simulink model "fault_predictor"  (R2024b)
settings: Solver=FixedStepDiscrete  StartTime=0.0  StopTime=T_stop  FixedStep=0.1  RelTol=1e-3
undefined symbols (not defined in the file): fp_thresholds
settings Model: Creator=rayen  LastModifiedBy=rayen
settings OptimizationCC: DefaultParameterBehavior=Inlined  EnhancedBackFolding=on  PassReuseOutputArgsAs=Individual arguments  ZeroExternalMemoryAtStartup=off  ZeroInternalMemoryAtStartup=off  OptimizeBlockOrder=speed  DifferentSizesBufferReuse=on  OptimizationCustomize=off  EfficientTunableParamExpr=on
settings DebuggingCC: ParameterTunabilityLossMsg=error
settings HardwareCC: TargetBitPerPointer=64  TargetBitPerSizeT=64  TargetBitPerPtrDiffT=64  TargetLargestAtomicFloat=Float  TargetIntDivRoundTo=Zero  TargetEndianess=LittleEndian  TargetWordSize=64  TargetHWDeviceType=Intel->x86-64 (Windows64)  ProdEqTarget=off
settings SFSimCC: MATLABDynamicMemAlloc=off  SimTargetLang=C++
settings RTWCC: Description=Embedded Coder  SystemTargetFile=ert.tlc  TemplateMakefile=ert_default_tmf
settings CodeAppCC: ForceParamTrailComments=on  IgnoreCustomStorageClasses=off  OperatorAnnotations=on  SimulinkDataObjDesc=on  SFDataObjDesc=on  InsertBlockDesc=on
settings ERTTargetCC: TargetLangStandard=C99 (ISO)  GenerateSampleERTMain=on  ERTCustomFileTemplate=example_file_process.tlc

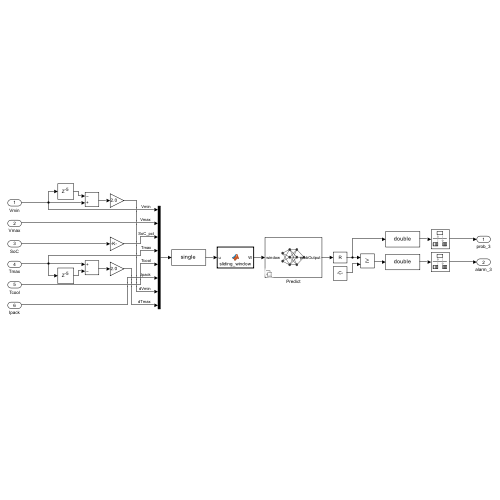
[thumbnail: Simulink's stored preview of the top-level diagram]
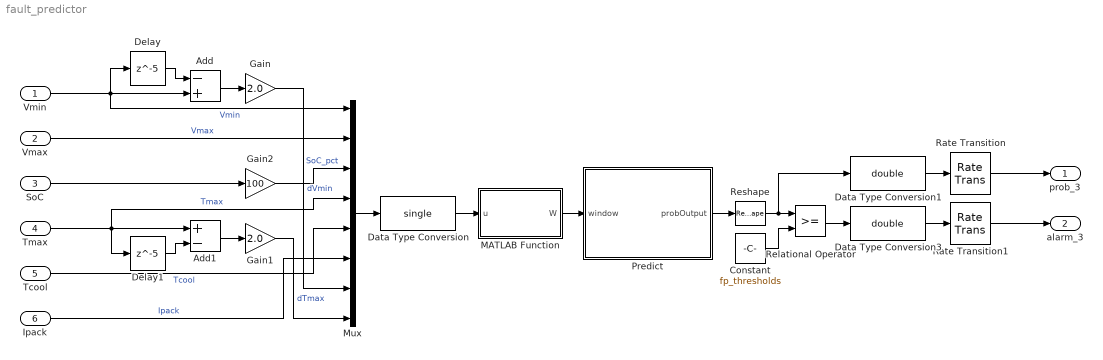
== system fault_predictor ==
  Vmin : Inport  SampleTime=0.1
  Vmax : Inport  Port=2  SampleTime=0.1
  SoC : Inport  Port=3  SampleTime=0.1
  Tmax : Inport  Port=4  SampleTime=0.1
  Tcool : Inport  Port=5  SampleTime=0.1
  Ipack : Inport  Port=6  SampleTime=0.1
  Add : Sum  Inputs=-+
  Add1 : Sum  Inputs=+-
  Constant : Constant  Value=fp_thresholds  OutDataTypeStr=single
  Data Type Conversion : DataTypeConversion  OutDataTypeStr=single  SaturateOnIntegerOverflow=off  RndMeth=Floor
  Data Type Conversion1 : DataTypeConversion  OutDataTypeStr=double  SaturateOnIntegerOverflow=off  RndMeth=Floor
  Data Type Conversion3 : DataTypeConversion  OutDataTypeStr=double  SaturateOnIntegerOverflow=off  RndMeth=Floor
  Delay : Delay  DelayLength=5  SampleTime=0.1
  Delay1 : Delay  DelayLength=5  SampleTime=0.1
  Gain : Gain  Gain=2.0
  Gain1 : Gain  Gain=2.0
  Gain2 : Gain  Gain=100
  MATLAB Function : MATLAB Function  TreatAsAtomicUnit=on
  Mux : Mux  Inputs=8
  Predict : Subsystem  Variant=on  VariantControl=Predict  AllowZeroVariantControls=on
  Rate Transition : RateTransition  OutPortSampleTime=0.1
  Rate Transition1 : RateTransition  OutPortSampleTime=0.1
  Relational Operator : RelationalOperator  OutDataTypeStr=boolean  RndMeth=Simplest  InputSameDT=off
  Reshape : Reshape  OutputDimensionality=Customize  OutputDimensions=[3 1]
  prob_3 : Outport
  alarm_3 : Outport  Port=2
  wires:
  Add/1 -> Gain/1
  Vmin/1 -> Mux/1, Delay/1, Add/2  "Vmin"
  Delay/1 -> Add/1
  Add1/1 -> Gain1/1
  Tmax/1 -> Mux/4, Delay1/1, Add1/1  "Tmax"
  Delay1/1 -> Add1/2
  SoC/1 -> Gain2/1
  Vmax/1 -> Mux/2  "Vmax"
  Gain2/1 -> Mux/3  "SoC_pct"
  Tcool/1 -> Mux/5  "Tcool"
  Gain/1 -> Mux/7  "dVmin"
  Gain1/1 -> Mux/8  "dTmax"
  Ipack/1 -> Mux/6  "Ipack"
  Mux/1 -> Data Type Conversion/1
  Data Type Conversion/1 -> MATLAB Function/1(u)
  Rate Transition/1 -> prob_3/1
  Rate Transition1/1 -> alarm_3/1
  Reshape/1 -> Data Type Conversion1/1, Relational Operator/1
  Constant/1 -> Relational Operator/2
  Relational Operator/1 -> Data Type Conversion3/1
  Data Type Conversion3/1 -> Rate Transition1/1
  Data Type Conversion1/1 -> Rate Transition/1
  MATLAB Function/1(W) -> Predict/1(window)
  Predict/1(probOutput) -> Reshape/1

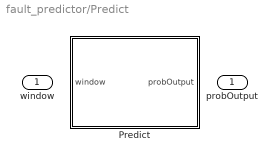
== system fault_predictor/Predict ==
  window : Inport
  Predict : Subsystem  VariantControl=true  mask(Predict){Network=Network from MAT-file, NetworkFunction=squeezenet, NetworkFilePath=C:\Users\rayen\Desktop\bms-engineering-assistant\ai\fault_prediction\inference\fault_predictor.mat, MiniBatchSize=1, InputDataFormats={'window', 'TCB';}, Predictions=on, Activations={}, ForceInterpretedSim=off, EnableDLNetwork=on, LastKnownNetworkFilePath='C:\Users\rayen\Desktop\bms-engineering-assistant\ai\fault_prediction\inference\fault_predictor.mat', LastKnownNetworkTimeStamp=740105.90783564816229045391082763671875}
      mask prompts: Network "deep_blocks:common:Network"; NetworkFunction "deep_blocks:common:MatlabFunction"; NetworkFilePath "deep_blocks:common:FilePath"; MiniBatchSize "deep_blocks:common:MiniBatchSize"; InputDataFormats "deep_blocks:predict:InputDataFormats"; Predictions "deep_blocks:common:Predictions"; Activations "deep_blocks:predict:Activations"; ForceInterpretedSim "deep_blocks:common:ForceInterpretedSim"
      mask help: deep_blocks:predict:Description
      mask init:
      | deep.blocks.internal.configureDeepNetwork(...
      |     gcb, ...
      |     bdroot, ...
      |     Network, ...
      |     NetworkFilePath, ...
      |     NetworkFunction, ...
      |     MiniBatchSize, ...
      |     logical(Predictions), ...
      |     InputDataFormats, ...
      |     Activations, ...
      |     logical(ForceInterpretedSim));
      mask Help: helpview('deeplearning', 'nnet_model_predict')
      mask TypeOptions Network: deep_blocks:common:NetworkFromMatFile | deep_blocks:common:NetworkFromFunction | squeezenet
      mask Callback Network:
      | deep.blocks.internal.setNetworkSelectVisibility(gcb);
      | deep.blocks.internal.setDlNetworkOptionsVisibility(gcb);
      | deep.blocks.internal.setActivations(gcb);
      mask Callback NetworkFunction:
      | deep.blocks.internal.setDlNetworkOptionsVisibility(gcb);
      | deep.blocks.internal.setActivations(gcb);
      mask Callback NetworkFilePath:
      | deep.blocks.internal.setDlNetworkOptionsVisibility(gcb);
      | deep.blocks.internal.setActivations(gcb);
      mask TypeOptions Activations: window | lstm | dense | relu | head
      mask DialogControl Network Prompt: Network:
      mask DialogControl NetworkFunction Prompt: MATLAB function:
      mask DialogControl NetworkFilePath Prompt: File path:
      mask DialogControl BrowseButton Prompt: deep_blocks:common:Browse
      mask DialogControl BrowseButton Callback: deep.blocks.internal.handleBrowseButtonClick(gcb);
      mask DialogControl MiniBatchSize Prompt: Mini-batch size:
      mask DialogControl InputDataFormats Prompt: Input data formats:
      mask DialogControl OutputsContainer Prompt: deep_blocks:common:Outputs
      mask DialogControl ActivationsContainer Prompt: deep_blocks:predict:Activations
      mask DialogControl HiddenContainer Prompt: Hidden Parameters
      mask DialogControl ForceInterpretedSim Prompt: Force interpreted simulation
  probOutput : Outport

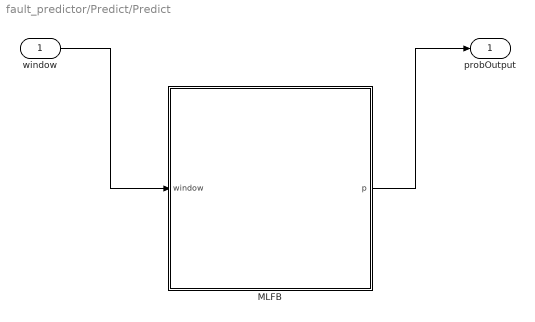
== system fault_predictor/Predict/Predict ==
  window : Inport
  MLFB : MATLAB Function  TreatAsAtomicUnit=on
  probOutput : Outport
  wires:
  window/1 -> MLFB/1(window)
  MLFB/1(p) -> probOutput/1

== matlab function fault_predictor/MATLAB Function ==
  data: u input; W output
function W = sliding_window(u)
%#codegen
persistent buf
if isempty(buf)
    buf = zeros(8, 50, 'single');
end
buf = [buf(:, 2:end), single(u(:))];
W = buf;
end

== matlab function fault_predictor/Predict/Predict/MLFB ==
  data: window input; p output
function p = deepNetwork(window)
%#codegen
% Stateful LSTM (hand-coded, 1 timestep/step). Same trained weights as the
% dlnetwork in fault_predictor.mat (max diff ~7e-9, single precision).
persistent w h c
if isempty(w)
    w = coder.load('C:\\Users\\rayen\\Desktop\\bms-engineering-assistant\\model\\fault_predictor\\inference\\fault_predictor_weights.mat');
    h = zeros(32, 1, 'single');
    c = zeros(32, 1, 'single');
end
% latest sample only; the LSTM state remembers the rest
u  = single(window(:, end));
x  = (u - w.norm_mean) ./ w.norm_std;
% LSTM gates: rows 1:32=i, 33:64=f, 65:96=g, 97:128=o (MATLAB convention)
z  = w.Wi * x + w.Wr * h + w.bL;
ig = single(1) ./ (single(1) + exp(-z(1:32)));
fg = single(1) ./ (single(1) + exp(-z(33:64)));
gg = tanh(z(65:96));
og = single(1) ./ (single(1) + exp(-z(97:128)));
c  = fg .* c + ig .* gg;
h  = og .* tanh(c);
% dense -> relu -> dense -> sigmoid
y1 = w.Wfc1 * h + w.bfc1;
y1 = max(y1, single(0));
y2 = w.Wfc2 * y1 + w.bfc2;
p  = single(1) ./ (single(1) + exp(-y2));
end
